simulink model "labc2"  (R2021b)
settings: Solver=FixedStepDiscrete  StartTime=0.0  StopTime=1e-4  FixedStep=50e-9  RelTol=1e-3
undefined symbols (not defined in the file): xc7k160tfbg676
libraries: hdlBasic x45, vmcUtilities x1
settings Model: Creator=Abdel  LastModifiedBy=Abdel

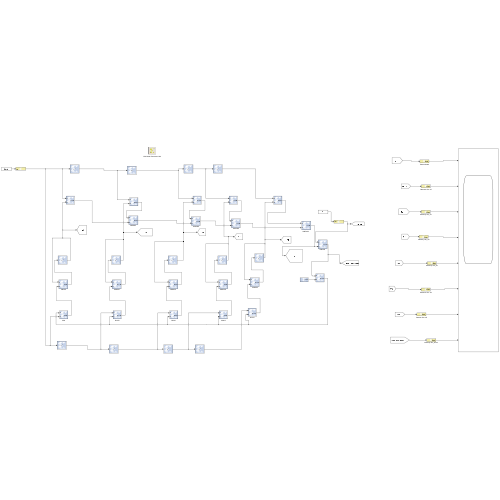
[thumbnail: Simulink's stored preview of the top-level diagram]
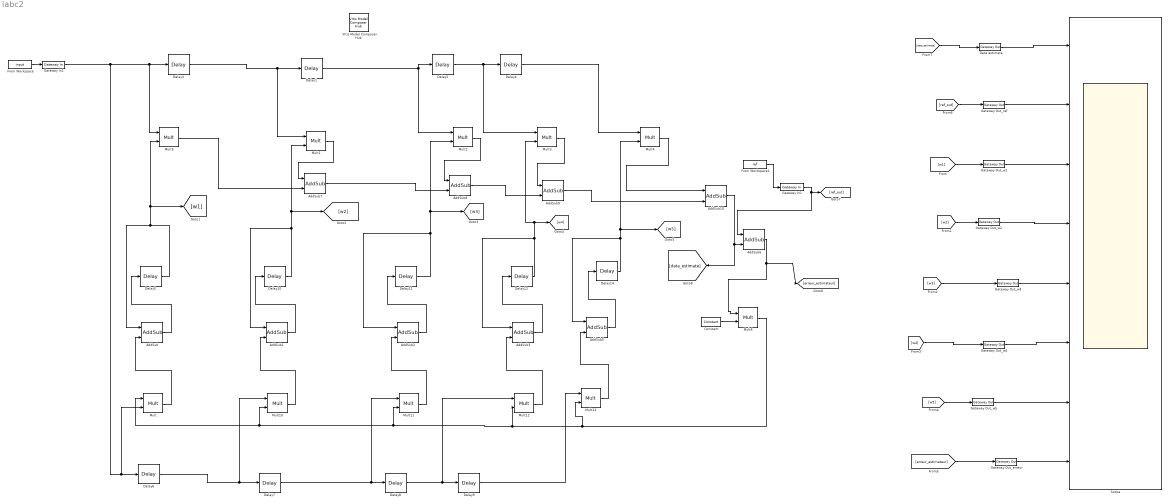
== system labc2 ==
  AddSub{,1..3,5,7..10} (9 alike) : hdlBasic/AddSub  mode=Addition  use_carryin=off  use_carryout=off  en=off  latency=0  precision=User Defined  arith_type="Signed  (2's comp)"  n_bits=16  bin_pt=14  quantization="Round  (unbiased: +/- Inf)"  overflow=Saturate  use_behavioral_HDL=off  hw_selection=Fabric  pipelined=off  XmcBlockStatus=1  maskContainerNames=tabcontainer1  block_type=addsub  block_config=sysgen:Addsub_config
  AddSub6 : hdlBasic/AddSub  mode=Subtraction  use_carryin=off  use_carryout=off  en=off  latency=0  precision=User Defined  arith_type="Signed  (2's comp)"  n_bits=16  bin_pt=14  quantization="Round  (unbiased: +/- Inf)"  overflow=Saturate  use_behavioral_HDL=off  hw_selection=Fabric  pipelined=off  XmcBlockStatus=1  maskContainerNames=tabcontainer1  block_type=addsub  block_config=sysgen:Addsub_config
  Constant : hdlBasic/Constant  const=0.25  gui_display_data_type=Fixed-point  arith_type=Signed (2's comp)  n_bits=16  bin_pt=14  preci_type=Single  exp_width=8  frac_width=24  explicit_period=on  period=50e-9  XmcBlockStatus=1  maskContainerNames=tabcontainer1  block_type=constant  block_config=sysgen:Constant_config
  Data estimate : hdlBasic/Gateway Out  inherit_from_input=off  hdl_port=on  rows=1  columns=1  UseAsDAC=off  DACChannel='1'  interface=None  automatic_assignment=on  address_offset=hex2dec('00')  intf_name=''  intf_description=''  timing_constraint=None  locs_specified=off  LOCs={}  io_standard={}  XmcBlockStatus=1  maskContainerNames=group4  block_type=gatewayout  block_config=sysgen:gateway_out_config  block_width_w=590  block_height_w=620  block_width=620  block_height=750
  Delay{1..12,14} (13 alike) : hdlBasic/Delay  rst=off  en=off  latency=1  reg_retiming=off  XmcBlockStatus=1  maskContainerNames=group1  block_type=delay  block_config=sysgen:Delay_config
  From Workspace : FromWorkspace  VariableName=input  SampleTime=-1  ZeroCross=off  OutputAfterFinalValue=Holding final value
  From Workspace1 : FromWorkspace  VariableName=ref  SampleTime=-1  ZeroCross=off  OutputAfterFinalValue=Holding final value
  Gateway In1 : hdlBasic/Gateway In  gui_display_data_type=Fixed-point  arith_type=Signed (2's comp)  n_bits=16  bin_pt=14  preci_type=Single  exp_width=8  frac_width=24  rows=1  columns=1  quantization="Round  (unbiased: +/- Inf)"  overflow=Saturate  period=50e-9  UseAsADC=off  ADCChannel='1'  interface=None  automatic_assignment=on  address_offset=hex2dec('00')  intf_name=''  intf_description=''  default_value=0  timing_constraint=None  locs_specified=off  LOCs={}  io_standard={}  inherit_from_input=off  hdl_port=on  XmcBlockStatus=1  maskContainerNames=group4  block_type=gatewayin  block_config=sysgen:gateway_in_config  block_width_w=590  block_height_w=620  block_width=640  block_height=850
  Gateway In2 : hdlBasic/Gateway In  gui_display_data_type=Fixed-point  arith_type=Signed (2's comp)  n_bits=16  bin_pt=14  preci_type=Single  exp_width=8  frac_width=24  rows=1  columns=1  quantization="Round  (unbiased: +/- Inf)"  overflow=Saturate  period=50e-9  UseAsADC=off  ADCChannel='1'  interface=None  automatic_assignment=on  address_offset=hex2dec('00')  intf_name=''  intf_description=''  default_value=0  timing_constraint=None  locs_specified=off  LOCs={}  io_standard={}  inherit_from_input=off  hdl_port=on  XmcBlockStatus=1  maskContainerNames=group4  block_type=gatewayin  block_config=sysgen:gateway_in_config  block_width_w=590  block_height_w=620  block_width=640  block_height=850
  Gateway Out_erreur : hdlBasic/Gateway Out  inherit_from_input=off  hdl_port=on  rows=1  columns=1  UseAsDAC=off  DACChannel='1'  interface=None  automatic_assignment=on  address_offset=hex2dec('00')  intf_name=''  intf_description=''  timing_constraint=None  locs_specified=off  LOCs={}  io_standard={}  XmcBlockStatus=1  maskContainerNames=group4  block_type=gatewayout  block_config=sysgen:gateway_out_config  block_width_w=590  block_height_w=620  block_width=620  block_height=750
  Gateway Out_ref : hdlBasic/Gateway Out  inherit_from_input=off  hdl_port=on  rows=1  columns=1  UseAsDAC=off  DACChannel='1'  interface=None  automatic_assignment=on  address_offset=hex2dec('00')  intf_name=''  intf_description=''  timing_constraint=None  locs_specified=off  LOCs={}  io_standard={}  XmcBlockStatus=1  maskContainerNames=group4  block_type=gatewayout  block_config=sysgen:gateway_out_config  block_width_w=590  block_height_w=620  block_width=620  block_height=750
  Gateway Out_w{1..5} (5 alike) : hdlBasic/Gateway Out  inherit_from_input=off  hdl_port=on  rows=1  columns=1  UseAsDAC=off  DACChannel='1'  interface=None  automatic_assignment=on  address_offset=hex2dec('00')  intf_name=''  intf_description=''  timing_constraint=None  locs_specified=off  LOCs={}  io_standard={}  XmcBlockStatus=1  maskContainerNames=group4  block_type=gatewayout  block_config=sysgen:gateway_out_config  block_width_w=590  block_height_w=620  block_width=620  block_height=750
  Mult{,1..6,10..13} (11 alike) : hdlBasic/Mult  precision=User Defined  arith_type="Signed  (2's comp)"  n_bits=16  bin_pt=14  quantization="Round  (unbiased: +/- Inf)"  overflow=Saturate  en=off  latency=0  use_behavioral_HDL=off  opt=Speed  use_embedded=on  optimum_pipeline=off  pipeline=on  use_rpm=on  placement_style=Triangular  XmcBlockStatus=1  maskContainerNames=group1  block_type=mult  block_config=sysgen:Mult_config
  Scope : Scope  NumInputPorts=8
  Vitis Model Composer Hub : vmcUtilities/Vitis Model Composer Hub  Tag=genX  CodeGeneration=off  SubsystemName=<enter or select subsystem name>  TargetDirectory=./code  ExportType=HLS C++ code  IpVendor=xilinx.com  IpLibrary=hls  IpVersion=1.0  IpHWLanguage=Verilog  AieCompilerOptions={}  CreateTestbench=off  TestbenchStackSize=10  RunAieSim=off  AieSimTimeout=50000  RunAieSimProfiling=off  LaunchVitisAnalyzer=off  PlotOutput=off  RunX86Sim=off  X86SimTimeout=10  GenHwImage=off  PlatformType=Not Specified  HwSystemType=Baremetal  HwValidationTarget=hw  ProjDevice=xc7k160tfbg676-3  ProjDevicePart=xc7k160tfbg676-3  SamplePeriod=-1  ClockFrequency=200  DataPathParallelism=1  xilinxfamily=kintex7  part=xc7k160t  speed=-3  package=fbg676  directory=./netlist  testbench=off  incr_netlist=off  synthesis_tool=Vivado  clock_wrapper=Clock Enables  dbl_ovrd=According to Block Masks  dcm_input_clock_period=10  sysclk_period=50  simulink_period=50e-9  eval_field=0
  wires:
  Delay3/1 -> Mult1/1, Delay1/1
  Delay1/1 -> Delay2/1, Mult2/1
  Delay2/1 -> Mult3/1, Delay4/1
  Delay4/1 -> Mult4/1
  Mult1/1 -> AddSub7/1
  Mult2/1 -> AddSub8/1
  Mult3/1 -> AddSub9/1
  Mult4/1 -> AddSub10/1
  Mult5/1 -> AddSub7/2
  AddSub7/1 -> AddSub8/2
  AddSub8/1 -> AddSub9/2
  AddSub9/1 -> AddSub10/2
  AddSub/1 -> Delay5/1
  Mult/1 -> AddSub/2
  Delay6/1 -> Mult10/1, Delay7/1
  Delay7/1 -> Mult11/1, Delay8/1
  AddSub1/1 -> Delay10/1
  Mult10/1 -> AddSub1/2
  AddSub2/1 -> Delay11/1
  Mult11/1 -> AddSub2/2
  AddSub3/1 -> Delay12/1
  Mult12/1 -> AddSub3/2
  AddSub6/1 -> Mult6/1, [erreur_estimateur]
  Delay5/1 -> Mult5/2, [w1], AddSub/1
  Delay10/1 -> Mult1/2, [w2], AddSub1/1
  Delay11/1 -> Mult2/2, [w3], AddSub2/1
  Delay12/1 -> Mult3/2, [w4], AddSub3/1
  Mult6/1 -> Mult13/2, Mult12/2, Mult/1, Mult10/2, Mult11/2
  Delay9/1 -> Mult13/1
  Mult13/1 -> AddSub5/2
  Delay14/1 -> Mult4/2, [w5], AddSub5/1
  AddSub5/1 -> Delay14/1
  Delay8/1 -> Mult12/1, Delay9/1
  Constant/1 -> Mult6/2
  AddSub10/1 -> AddSub6/2, [data_estimate]
  Gateway In1/1 -> AddSub6/1, [ref_out]
  [erreur_estimateur] -> Gateway Out_erreur/1
  [w5] -> Gateway Out_w5/1
  [w4] -> Gateway Out_w4/1
  [w3] -> Gateway Out_w3/1
  [w2] -> Gateway Out_w2/1
  [w1] -> Gateway Out_w1/1
  Gateway Out_w1/1 -> Scope/3
  Gateway Out_w2/1 -> Scope/4
  Gateway Out_w3/1 -> Scope/5
  Gateway Out_w4/1 -> Scope/6
  Gateway Out_w5/1 -> Scope/7
  Gateway In2/1 -> Mult/2, Delay6/1, Mult5/1, Delay3/1
  From Workspace/1 -> Gateway In2/1
  From Workspace1/1 -> Gateway In1/1
  [ref_out] -> Gateway Out_ref/1
  Gateway Out_ref/1 -> Scope/2
  Gateway Out_erreur/1 -> Scope/8
  Data estimate/1 -> Scope/1
  [data_estimate] -> Data estimate/1
